simulink model "mymodel_v2"  (R2020b)
settings: Solver=FixedStepAuto  StartTime=0  StopTime=0.5  FixedStep=Ts  RelTol=1e-3
values from neighbouring files (symbols this model uses):
  Ts = 1/Fs    (= 0.001)    [Test.m]
  Wbase = Fbase*2*pi    (= 314.159265359)    [Test.m]
libraries: powerlib x9, SimplusGT x4
settings Model: Creator=admin_user  LastModifiedBy=admin_user

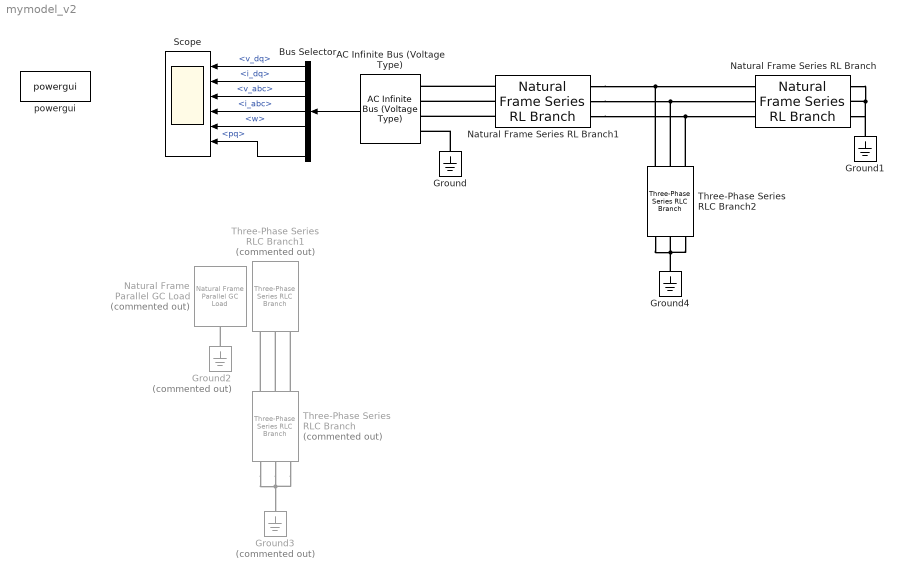
== system mymodel_v2 ==
  AC Infinite Bus (Voltage Type) : SimplusGT/AC Infinite Bus (Voltage Type)  Ts=Ts  Sbase=1  Vbase=1  Wbase=Wbase  vd=1  vq=0  theta0=0  w=Wbase  R=1e-30
  Bus Selector : BusSelector  OutputSignals=v_dq,i_dq,v_abc,i_abc,w,theta,pq
  Ground : powerlib/Elements/Ground  LConnTagsString=a
  Ground1 : powerlib/Elements/Ground  LConnTagsString=a
  Ground2 : powerlib/Elements/Ground  Commented=on  LConnTagsString=a
  Ground3 : powerlib/Elements/Ground  Commented=on  LConnTagsString=a
  Ground4 : powerlib/Elements/Ground  LConnTagsString=a
  Natural Frame Parallel GC Load : SimplusGT/Natural Frame Parallel GC Load  Commented=on  Ts=Ts  G=1e-6  C=0
  Natural Frame Series RL Branch : SimplusGT/Natural Frame Series RL Branch  Ts=Ts  R=1/5  L=1/Wbase
  Natural Frame Series RL Branch1 : SimplusGT/Natural Frame Series RL Branch  Ts=Ts  R=1/5  L=1/Wbase
  Scope : Scope  NumInputPorts=6
  Three-Phase Series RLC Branch : powerlib/Elements/Three-Phase Series RLC Branch  Commented=on  LConnTagsString=A|B|C  RConnTagsString=A|B|C  BranchType=C  Resistance=1  Inductance=1e-3  Capacitance=1/Wbase  Measurements=None
  Three-Phase Series RLC Branch1 : powerlib/Elements/Three-Phase Series RLC Branch  Commented=on  LConnTagsString=A|B|C  RConnTagsString=A|B|C  BranchType=R  Resistance=1e-3  Inductance=1e-3  Capacitance=1/Wbase  Measurements=None
  Three-Phase Series RLC Branch2 : powerlib/Elements/Three-Phase Series RLC Branch  LConnTagsString=A|B|C  RConnTagsString=A|B|C  BranchType=R  Resistance=1e3  Inductance=1e-3  Capacitance=1/Wbase  Measurements=None
  powergui : powerlib/powergui  Priority=1  SimulationMode=Discrete  SampleTime=Ts  frequency=60  Iterations=50  frequencyindice=0  Pbase=100e6  ErrMax=1e-4  UnitsV=kV  UnitsW=MW  buscounter=0  FunctionMessages=off  echomessages=off  EnableUseOfTLC=off  CurrentSourceSwitches=off  DisableSnubberDevices=off  DisableRonSwitches=off  DisableVfSwitches=off  DisplayEquations=off  AutomaticDiscreteSolvers=off  SolverType=Tustin/Backward Euler (TBE)  Interpol=off  ExternalGateDelay=off  methode=off  Ts=100  x0status=blocks  SPID=on  SwTol=0  HookPort=off  NonlinearTolerance=1e-4  nMaxIteration=100  ContinueOnMaxIteration=off  RestoreLinks=warning  ResistiveCurrentMeasurement=off  Frange=[0:2:500]  Ylog=off  Xlog=on  ShowGrid=off  save=off  variable=ZData  structure=0  ZoomFFT=off  StartTime=0.0  cycles=1  DisplayStyle=1  fundamental=60  FreqAxis=off  MaxFrequency=1000  frequencyindicesteady=1  RmsSteady=1  display=off
  wires:
  AC Infinite Bus (Voltage Type)/1 -> Bus Selector/1
  Bus Selector/1 -> Scope/1  "<v_dq>"
  Bus Selector/2 -> Scope/2  "<i_dq>"
  Bus Selector/3 -> Scope/3  "<v_abc>"
  Bus Selector/4 -> Scope/4  "<i_abc>"
  Bus Selector/5 -> Scope/5  "<w>"
  Bus Selector/7 -> Scope/6  "<pq>"
  connections:
  Natural Frame Series RL Branch/RConn1 -- Ground1/LConn1 -- Natural Frame Series RL Branch/RConn3 -- Natural Frame Series RL Branch/RConn2
  Ground/LConn1 -- AC Infinite Bus (Voltage Type)/LConn4
  Natural Frame Series RL Branch1/RConn1 -- Three-Phase Series RLC Branch2/LConn1 -- Natural Frame Series RL Branch/LConn1
  Natural Frame Series RL Branch1/RConn3 -- Three-Phase Series RLC Branch2/LConn3 -- Natural Frame Series RL Branch/LConn3
  Natural Frame Series RL Branch1/RConn2 -- Three-Phase Series RLC Branch2/LConn2 -- Natural Frame Series RL Branch/LConn2
  Natural Frame Series RL Branch1/LConn1 -- AC Infinite Bus (Voltage Type)/LConn1
  Natural Frame Series RL Branch1/LConn2 -- AC Infinite Bus (Voltage Type)/LConn2
  Natural Frame Series RL Branch1/LConn3 -- AC Infinite Bus (Voltage Type)/LConn3
  Ground2/LConn1 -- Natural Frame Parallel GC Load/LConn1
  Three-Phase Series RLC Branch/RConn2 -- Three-Phase Series RLC Branch/RConn3 -- Three-Phase Series RLC Branch/RConn1 -- Ground3/LConn1
  Three-Phase Series RLC Branch/LConn1 -- Three-Phase Series RLC Branch1/RConn1
  Three-Phase Series RLC Branch/LConn2 -- Three-Phase Series RLC Branch1/RConn2
  Three-Phase Series RLC Branch/LConn3 -- Three-Phase Series RLC Branch1/RConn3
  Ground4/LConn1 -- Three-Phase Series RLC Branch2/RConn3 -- Three-Phase Series RLC Branch2/RConn1 -- Three-Phase Series RLC Branch2/RConn2
